simulink model "EV_simulation_motor"  (R2024b)
settings: Solver=VariableStepAuto  StartTime=0.0  StopTime=10.0  RelTol=1e-3
settings Model: Creator=brain  LastModifiedBy=brain

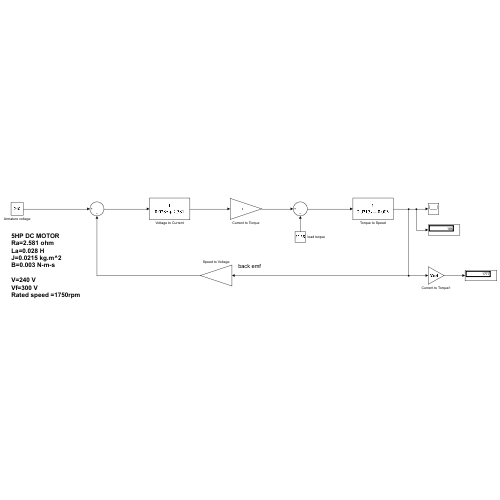
[thumbnail: Simulink's stored preview of the top-level diagram]
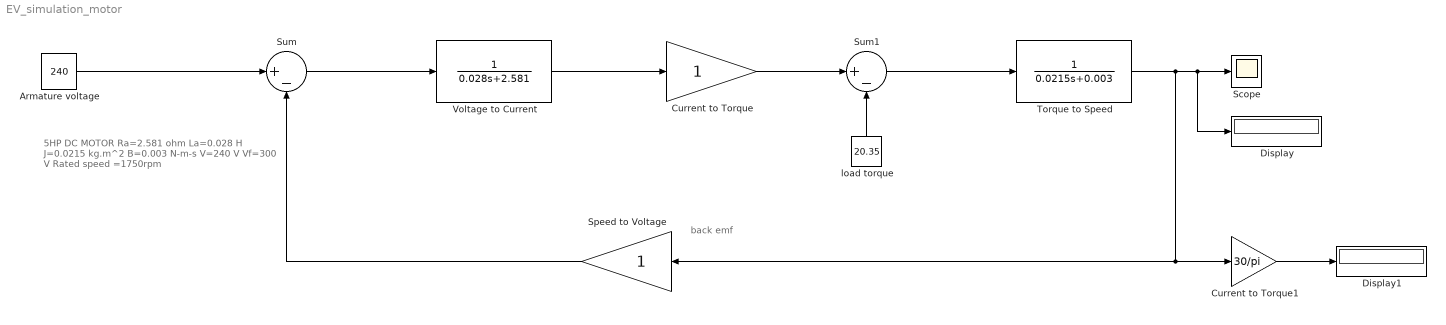
== system EV_simulation_motor ==
  note: back emf
  note: 5HP DC MOTOR
      | Ra=2.581 ohm
      | La=0.028 H
      | J=0.0215 kg.m^2
      | B=0.003 N-m-s
      |
      | V=240 V
      | Vf=300 V
      | Rated speed =1750rpm
  Armature voltage : Constant  Value=240
  Current to Torque : Gain
  Current to Torque1 : Gain  Gain=30/pi
  Display : Display
  Display1 : Display
  Scope : Scope
  Speed to Voltage : Gain
  Sum : Sum  Inputs=|+-
  Sum1 : Sum  Inputs=|+-
  Torque to Speed : TransferFcn  Denominator=[0.0215 0.003]
  Voltage to Current : TransferFcn  Denominator=[0.028 2.581]
  load torque : Constant  Value=20.35
  wires:
  Sum/1 -> Voltage to Current/1
  Voltage to Current/1 -> Current to Torque/1
  Current to Torque/1 -> Sum1/1
  Sum1/1 -> Torque to Speed/1
  load torque/1 -> Sum1/2
  Speed to Voltage/1 -> Sum/2
  Armature voltage/1 -> Sum/1
  Torque to Speed/1 -> Display/1, Scope/1, Speed to Voltage/1, Current to Torque1/1
  Current to Torque1/1 -> Display1/1
